simulink model "calc"  (R2021a)
settings: Solver=FixedStepDiscrete  StartTime=0.0  StopTime=10.0  RelTol=1e-3  EnableMultiTasking=on
libraries: simulink x2
settings Model: Creator=Dell  LastModifiedBy=Dell
settings DataIOCC: ReturnWorkspaceOutputs=off
settings OptimizationCC: DefaultParameterBehavior=Inlined  InlineInvariantSignals=on  EnableMemcpy=off  LifeSpan=1  EfficientTunableParamExpr=on
settings DebuggingCC: UnderspecifiedInitializationDetection=Classic  MergeDetectMultiDrivingBlocksExec=none  SFMachineParentedDataDiag=warning  ArithmeticOperatorsInVariantConditions=warning
settings ModelReferenceCC: PropagateSignalLabelsOutOfModel=off
settings SFSimCC: MATLABDynamicMemAlloc=off  CustomCodeUndefinedFunction=UseInterfaceOnly
settings RTWCC: SystemTargetFile=ert.tlc  GenCodeOnly=on  TemplateMakefile=ert_default_tmf  GenerateReport=on  IncludeHyperlinkInReport=on  LaunchReport=on  GenerateTraceInfo=on  GenerateTraceReport=on  GenerateTraceReportSl=on  GenerateTraceReportSf=on  GenerateTraceReportEml=on
settings CodeAppCC: ForceParamTrailComments=on  IgnoreCustomStorageClasses=off  OperatorAnnotations=on  SimulinkDataObjDesc=on  SFDataObjDesc=on  MATLABFcnDesc=on  InsertBlockDesc=on  StateflowObjectComments=on  MATLABSourceComments=on
settings ERTTargetCC: MultiwordLength=2048  GenerateSampleERTMain=on  InlinedParameterPlacement=NonHierarchical  ERTCustomFileTemplate=example_file_process.tlc

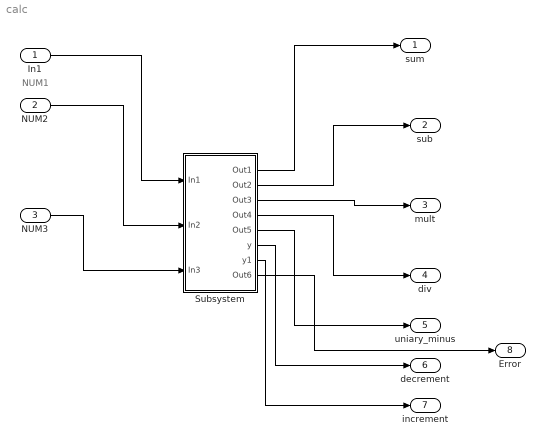
== system calc ==
  note: NUM1
  In1 : Inport
  NUM2 : Inport  Port=2
  NUM3 : Inport  Port=3
  Subsystem : Subsystem
  sum : Outport
  sub : Outport  Port=2
  mult : Outport  Port=3
  div : Outport  Port=4
  uniary_minus : Outport  Port=5
  decrement : Outport  Port=6
  increment : Outport  Port=7
  Error : Outport  Port=8
  wires:
  In1/1 -> Subsystem/1(In1)
  NUM2/1 -> Subsystem/2(In2)
  NUM3/1 -> Subsystem/3(In3)
  Subsystem/1(Out1) -> sum/1
  Subsystem/2(Out2) -> sub/1
  Subsystem/3(Out3) -> mult/1
  Subsystem/4(Out4) -> div/1
  Subsystem/5(Out5) -> uniary_minus/1
  Subsystem/6(y) -> decrement/1
  Subsystem/7(y1) -> increment/1
  Subsystem/8(Out6) -> Error/1

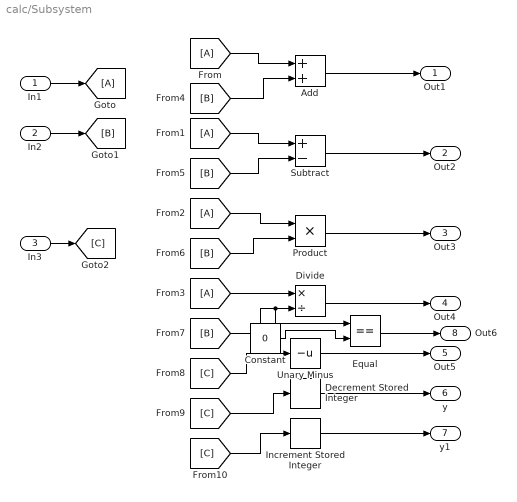
== system calc/Subsystem ==
  In1 : Inport
  In2 : Inport  Port=2
  In3 : Inport  Port=3
  Add : Sum
  Constant : Constant  Value=0
  Decrement Stored Integer : simulink/Additional Math & Discrete/Additional Math: Increment - Decrement/Decrement Stored Integer
      settings: SourceProductBaseCode=SL
  Divide : Product  Inputs=*/
  Equal : RelationalOperator  Operator===  OutDataTypeStr=boolean  RndMeth=Simplest
  Increment Stored Integer : simulink/Additional Math & Discrete/Additional Math: Increment - Decrement/Increment Stored Integer
  Product : Product
  Subtract : Sum  Inputs=+-
  Unary Minus : UnaryMinus
  Out1 : Outport
  Out2 : Outport  Port=2
  Out3 : Outport  Port=3
  Out4 : Outport  Port=4
  Out5 : Outport  Port=5
  y : Outport  Port=6
  y1 : Outport  Port=7
  Out6 : Outport  Port=8
  wires:
  Divide/1 -> Out4/1
  [B] -> Subtract/2
  [C] -> Decrement Stored Integer/1
  Unary Minus/1 -> Out5/1
  Decrement Stored Integer/1 -> y/1
  [A] -> Divide/1
  [A] -> Product/1
  Increment Stored Integer/1 -> y1/1
  [A] -> Add/1
  [A] -> Subtract/1
  [B] -> Add/2
  [C] -> Unary Minus/1
  [B] -> Equal/1, Divide/2
  [B] -> Product/2
  Product/1 -> Out3/1
  [C] -> Increment Stored Integer/1
  In2/1 -> [B]
  In1/1 -> [A]
  In3/1 -> [C]
  Add/1 -> Out1/1
  Subtract/1 -> Out2/1
  Constant/1 -> Equal/2
  Equal/1 -> Out6/1
